simulink library "singleTetherSpooling"  (R2018b)
settings: Solver=VariableStepAuto  StartTime=0.0  StopTime=10.0  RelTol=1e-3
undefined symbols (not defined in the file): altiMax, altiMin, ctrl, initializeBussesFromBlock, wnch
libraries: filteredPIDController_ul x2
settings Model: Creator=asiddiq2  LastModifiedBy=mcobb

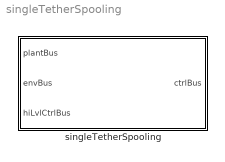
== system singleTetherSpooling ==
  singleTetherSpooling : Subsystem  LoadFcn=initializeBussesFromBlock(gcb)  InitFcn=initializeBussesFromBlock(gcb)  StartFcn=initializeBussesFromBlock(gcb)

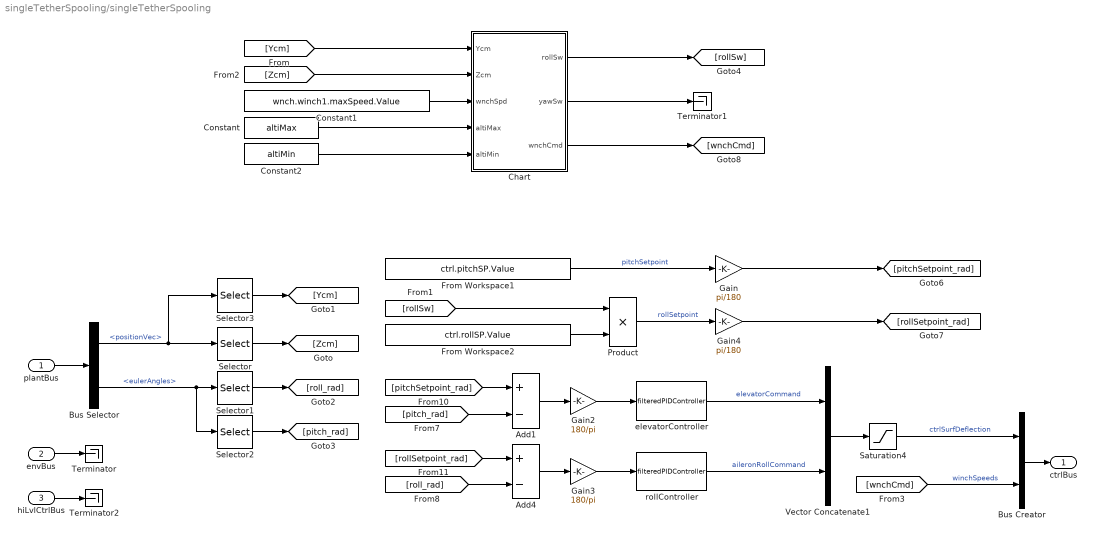
== system singleTetherSpooling/singleTetherSpooling ==
  plantBus : Inport  OutDataTypeStr=Bus: plantBus
  envBus : Inport  Port=2  OutDataTypeStr=Bus: envBus
  hiLvlCtrlBus : Inport  Port=3  OutDataTypeStr=Bus: hiLvlCtrlBus
  Add1 : Sum  Inputs=+-
  Add4 : Sum  Inputs=+-
  Bus Creator : BusCreator  Inputs=2  OutDataTypeStr=Bus: fltCtrlBus
  Bus Selector : BusSelector  OutputSignals=positionVec,eulerAngles
  Chart : Stateflow chart  TreatAsAtomicUnit=on
  Constant : Constant  Value=altiMax
  Constant1 : Constant  Value=wnch.winch1.maxSpeed.Value  VectorParams1D=off
  Constant2 : Constant  Value=altiMin
  From Workspace1 : FromWorkspace  VariableName=ctrl.pitchSP.Value  SampleTime=0
  From Workspace2 : FromWorkspace  VariableName=ctrl.rollSP.Value  SampleTime=0
  Gain : Gain  Gain=pi/180
  Gain2 : Gain  Gain=180/pi
  Gain3 : Gain  Gain=180/pi
  Gain4 : Gain  Gain=pi/180
  Product : Product
  Saturation4 : Saturate  UpperLimit=ctrl.outputSat.upperLimit.Value  LowerLimit=ctrl.outputSat.lowerLimit.Value
  Selector : Selector  InputPortWidth=3  IndexOptions=Index vector (dialog)  Indices=3  OutputSizes=1
  Selector1 : Selector  InputPortWidth=3  IndexOptions=Index vector (dialog)  Indices=1  OutputSizes=1
  Selector2 : Selector  InputPortWidth=3  IndexOptions=Index vector (dialog)  Indices=2  OutputSizes=1
  Selector3 : Selector  InputPortWidth=3  IndexOptions=Index vector (dialog)  Indices=2  OutputSizes=1
  Terminator : Terminator
  Terminator1 : Terminator
  Terminator2 : Terminator
  Vector Concatenate1 : Concatenate
  elevatorController : filteredPIDController_ul/filteredPIDController  kp=ctrl.elevators.kp.Value  ki=ctrl.elevators.ki.Value  kd=ctrl.elevators.kd.Value  Value=ctrl.elevators.tau.Value
  rollController : filteredPIDController_ul/filteredPIDController  kp=ctrl.ailerons.kp.Value  ki=ctrl.ailerons.ki.Value  kd=ctrl.ailerons.kd.Value  Value=ctrl.ailerons.tau.Value
  ctrlBus : Outport  OutDataTypeStr=Bus: fltCtrlBus
  wires:
  plantBus/1 -> Bus Selector/1
  Selector2/1 -> [pitch_rad]
  Gain/1 -> [pitchSetpoint_rad]
  Add4/1 -> Gain3/1
  Selector1/1 -> [roll_rad]
  Gain3/1 -> rollController/1
  Bus Selector/2 -> Selector2/1, Selector1/1  "<eulerAngles>"
  From Workspace1/1 -> Gain/1  "pitchSetpoint"
  Bus Creator/1 -> ctrlBus/1
  [pitchSetpoint_rad] -> Add1/1
  rollController/1 -> Vector Concatenate1/2  "aileronRollCommand"
  envBus/1 -> Terminator/1
  [roll_rad] -> Add4/2
  Vector Concatenate1/1 -> Saturation4/1
  Add1/1 -> Gain2/1
  Gain2/1 -> elevatorController/1
  Bus Selector/1 -> Selector3/1, Selector/1  "<positionVec>"
  elevatorController/1 -> Vector Concatenate1/1  "elevatorCommand"
  [rollSetpoint_rad] -> Add4/1
  Selector/1 -> [Zcm]
  Saturation4/1 -> Bus Creator/1  "ctrlSurfDeflection"
  [wnchCmd] -> Bus Creator/2  "winchSpeeds"
  [pitch_rad] -> Add1/2
  Chart/1(rollSw) -> [rollSw]
  [Ycm] -> Chart/1(Ycm)
  Constant1/1 -> Chart/3(wnchSpd)
  Chart/2(yawSw) -> Terminator1/1
  Selector3/1 -> [Ycm]
  [rollSw] -> Product/1
  Gain4/1 -> [rollSetpoint_rad]
  [Zcm] -> Chart/2(Zcm)
  Chart/3(wnchCmd) -> [wnchCmd]
  Constant/1 -> Chart/4(altiMax)
  Constant2/1 -> Chart/5(altiMin)
  From Workspace2/1 -> Product/2
  Product/1 -> Gain4/1  "rollSetpoint"
  hiLvlCtrlBus/1 -> Terminator2/1

== stateflow chart singleTetherSpooling/Chart ==
  state SpoolOut
    entry:
    wnchCmd = wnchSpd/4;
    rollSw = 1;
    yawSw = 0;
    during:
    wnchCmd = wnchSpd/4;
    rollSw = 1;
    yawSw = 0;
  state Spoolin
    entry:
    wnchCmd = -wnchSpd;
    rollSw = 0;
    yawSw = 1;
    during:
    wnchCmd = -wnchSpd;
    rollSw = 0;
    yawSw = 1;
  (default) -> SpoolOut
  SpoolOut -> Spoolin : [Zcm>altiMax && norm(Ycm)<0.5]
  Spoolin -> SpoolOut : [Zcm<altiMin]
  data: Ycm input; Zcm input; wnchSpd input; rollSw output; yawSw output; wnchCmd output; altiMax input; altiMin input
